simulink model "motorsetup"  (R2015b)
settings: Solver=VariableStepAuto  StartTime=0.0  StopTime=10.0  RelTol=1e-3
values from neighbouring files (symbols this model uses):
  Ra = 1/fit1.Coefficients.Estimate(2)    [parameterization.m]
undefined symbols (not defined in the file or in its folder): Kt
libraries: fl_lib x12, elec_lib x1
settings Model: Creator=thomas  LastModifiedBy=thomas

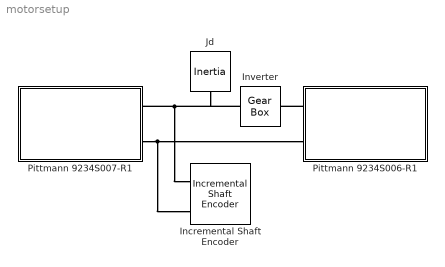
== system motorsetup ==
  Incremental Shaft Encoder : elec_lib/Sensors/Incremental Shaft Encoder  NPulse=500  Vm=5 V  angle0=0 deg
  Inverter : fl_lib/Mechanical/Mechanisms/Gear Box  ratio=-1  t_in_specify=off  t_in_priority=None  t_in=0 N*m  t_out_specify=off  t_out_priority=None  t_out=0 N*m
  Jd : fl_lib/Mechanical/Rotational Elements/Inertia  inertia=0.01 kg*m^2  w_specify=off  w_priority=None  w=0 rad/s  t_specify=off  t_priority=None  t=0 N*m
  Pittmann 9234S006-R1 : Subsystem
  Pittmann 9234S007-R1 : Subsystem
  connections:
  Inverter/LConn1 -- Jd/LConn1 -- Pittmann 9234S007-R1/RConn1 -- Incremental Shaft Encoder/LConn1
  Pittmann 9234S007-R1/RConn2 -- Incremental Shaft Encoder/LConn2 -- Pittmann 9234S006-R1/RConn2
  Pittmann 9234S006-R1/RConn1 -- Inverter/RConn1

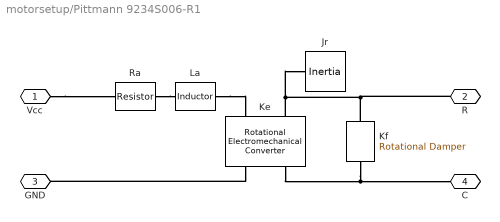
== system motorsetup/Pittmann 9234S006-R1 ==
  Jr : fl_lib/Mechanical/Rotational Elements/Inertia  inertia=Jr kg*m^2  w_specify=off  w_priority=None  w=0 rad/s  t_specify=off  t_priority=None  t=0 N*m
  Ke : fl_lib/Electrical/Electrical Elements/Rotational Electromechanical Converter  K=Kt V/(rad/s)  i_specify=off  i_priority=None  i=0 A  v_specify=off  v_priority=None  v=0 V  t_specify=off  t_priority=None  t=0 N*m  w_specify=off  w_priority=None  w=0 rad/s
  Kf : fl_lib/Mechanical/Rotational Elements/Rotational Damper  D=0.001 N*m/(rad/s)  w_specify=off  w_priority=None  w=0 rad/s  t_specify=off  t_priority=None  t=0 N*m
  La : fl_lib/Electrical/Electrical Elements/Inductor  l=L mH  r=0 Ohm  g=1e-9 1/Ohm  i_specify=off  i_priority=None  i=0 A  v_specify=off  v_priority=None  v=0 V  i_L_specify=off  i_L_priority=None  i_L=0 A
  Ra : fl_lib/Electrical/Electrical Elements/Resistor  R=Ra Ohm  i_specify=off  i_priority=None  i=0 A  v_specify=off  v_priority=None  v=0 V
  Vcc : PMIOPort  Port=1  Side=Left
  R : PMIOPort  Port=2  Side=Right
  GND : PMIOPort  Port=3  Side=Left
  C : PMIOPort  Port=4  Side=Right
  connections:
  Kf/LConn1 -- Ke/LConn2 -- Jr/LConn1 -- R/RConn1
  Ke/RConn2 -- Kf/RConn1 -- C/RConn1
  La/RConn1 -- Ke/LConn1
  Ke/RConn1 -- GND/RConn1
  Ra/RConn1 -- La/LConn1
  Vcc/RConn1 -- Ra/LConn1

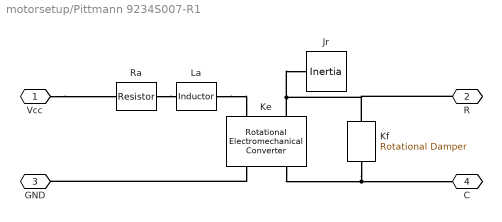
== system motorsetup/Pittmann 9234S007-R1 ==
  Jr : fl_lib/Mechanical/Rotational Elements/Inertia  inertia=Jr kg*m^2  w_specify=off  w_priority=None  w=0 rad/s  t_specify=off  t_priority=None  t=0 N*m
  Ke : fl_lib/Electrical/Electrical Elements/Rotational Electromechanical Converter  K=Kt V/(rad/s)  i_specify=off  i_priority=None  i=0 A  v_specify=off  v_priority=None  v=0 V  t_specify=off  t_priority=None  t=0 N*m  w_specify=off  w_priority=None  w=0 rad/s
  Kf : fl_lib/Mechanical/Rotational Elements/Rotational Damper  D=0.001 N*m/(rad/s)  w_specify=off  w_priority=None  w=0 rad/s  t_specify=off  t_priority=None  t=0 N*m
  La : fl_lib/Electrical/Electrical Elements/Inductor  l=L mH  r=0 Ohm  g=1e-9 1/Ohm  i_specify=off  i_priority=None  i=0 A  v_specify=off  v_priority=None  v=0 V  i_L_specify=off  i_L_priority=None  i_L=0 A
  Ra : fl_lib/Electrical/Electrical Elements/Resistor  R=Ra Ohm  i_specify=off  i_priority=None  i=0 A  v_specify=off  v_priority=None  v=0 V
  Vcc : PMIOPort  Port=1  Side=Left
  R : PMIOPort  Port=2  Side=Right
  GND : PMIOPort  Port=3  Side=Left
  C : PMIOPort  Port=4  Side=Right
  connections:
  Ke/LConn2 -- R/RConn1 -- Kf/LConn1 -- Jr/LConn1
  Kf/RConn1 -- C/RConn1 -- Ke/RConn2
  La/RConn1 -- Ke/LConn1
  Ke/RConn1 -- GND/RConn1
  Ra/RConn1 -- La/LConn1
  Vcc/RConn1 -- Ra/LConn1
